simulink model "calibrate_imu_2_2"  (R2021b)
settings: Solver=VariableStepAuto  StartTime=0.0  StopTime=10.0  RelTol=1e-3
undefined symbols (not defined in the file or in its folder): X, Y, Z
libraries: nesl_utility x16, sm_lib x9, robotcorelib x1, aerolibnav x1
(part 2 of 2)

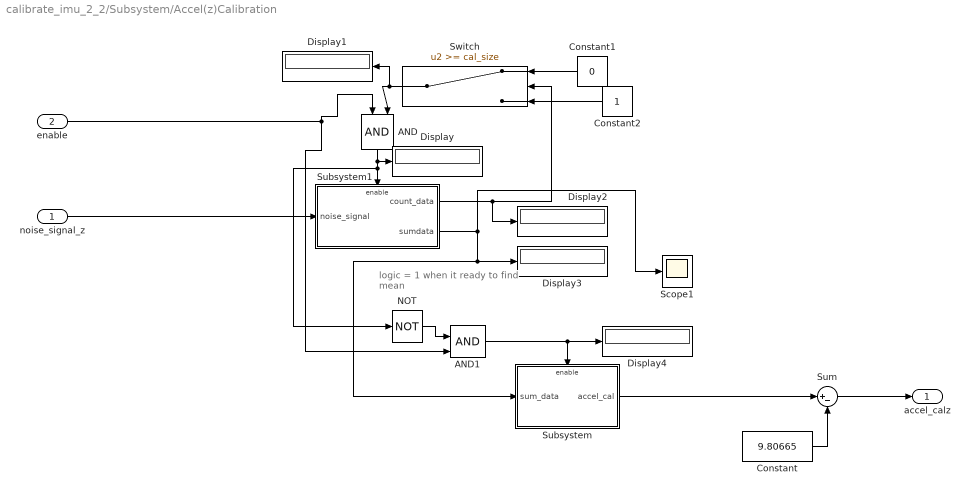
== system calibrate_imu_2_2/Subsystem/Accel(z)Calibration ==
  note: logic = 1 when it ready
      | to find mean
  noise_signal_z : Inport
  enable : Inport  Port=2
  AND : Logic  IconShape=distinctive  AllPortsSameDT=off  OutDataTypeStr=boolean
  AND1 : Logic  IconShape=distinctive  AllPortsSameDT=off  OutDataTypeStr=boolean
  Constant : Constant  Value=9.80665
  Constant1 : Constant  Value=0
  Constant2 : Constant
  Display{,1..4} (5 alike) : Display
  NOT : Logic  Operator=NOT  IconShape=distinctive  AllPortsSameDT=off  OutDataTypeStr=boolean
  Scope1 : Scope
  Subsystem : Subsystem
  Subsystem1 : Subsystem
  Sum : Sum  Inputs=|+-
  Switch : Switch  Threshold=cal_size
  accel_calz : Outport
  wires:
  Subsystem1/2(sumdata) -> Display3/1, Subsystem/1(sum_data), Scope1/1
  enable/1 -> AND/1, AND1/2
  Constant1/1 -> Switch/1
  Constant2/1 -> Switch/3
  Switch/1 -> Display1/1, AND/2
  AND/1 -> NOT/1, Subsystem1/Enable, Display/1
  NOT/1 -> AND1/1
  AND1/1 -> Subsystem/Enable, Display4/1
  Subsystem1/1(count_data) -> Switch/2, Display2/1
  noise_signal_z/1 -> Subsystem1/1(noise_signal)
  Sum/1 -> accel_calz/1
  Subsystem/1(accel_cal) -> Sum/1
  Constant/1 -> Sum/2

== system calibrate_imu_2_2/Gyro_Calibration/Gyro(x)Calibration/mean ==
  sum_data : Inport
  Enable : EnablePort
  Constant4 : Constant  Value=1000
  Divide : Product  Inputs=*/
  gyro_cal : Outport
  wires:
  Divide/1 -> gyro_cal/1  "gyro_cal"
  Constant4/1 -> Divide/2
  sum_data/1 -> Divide/1

== system calibrate_imu_2_2/Gyro_Calibration/Gyro(x)Calibration/sumdata ==
  noise_signal : Inport
  Enable : EnablePort
  Pulse Generator : DiscretePulseGenerator  PulseType=Time based  Period=sampleT  PulseWidth=5
  Subsystem : Subsystem
  count_data : Outport
  sumdata : Outport  Port=2
  wires:
  Pulse Generator/1 -> Subsystem/Trigger
  Subsystem/1(Out1) -> count_data/1
  Subsystem/2(Out2) -> sumdata/1
  noise_signal/1 -> Subsystem/1(noise signal)

== system calibrate_imu_2_2/Gyro_Calibration/Gyro(y)Calibration1/Subsystem ==
  sum_data : Inport
  Enable : EnablePort
  Constant4 : Constant  Value=1000
  Divide : Product  Inputs=*/
  gyro_cal : Outport
  wires:
  Divide/1 -> gyro_cal/1  "gyro_cal"
  Constant4/1 -> Divide/2
  sum_data/1 -> Divide/1

== system calibrate_imu_2_2/Gyro_Calibration/Gyro(y)Calibration1/Subsystem1 ==
  noise_signal : Inport
  Enable : EnablePort
  Pulse Generator : DiscretePulseGenerator  PulseType=Time based  Period=sampleT  PulseWidth=5
  Subsystem : Subsystem
  count_data : Outport
  sumdata : Outport  Port=2
  wires:
  Pulse Generator/1 -> Subsystem/Trigger
  Subsystem/1(Out1) -> count_data/1
  Subsystem/2(Out2) -> sumdata/1
  noise_signal/1 -> Subsystem/1(noise signal)

== system calibrate_imu_2_2/Gyro_Calibration/Gyro(z)Calibration2/Subsystem ==
  sum_data : Inport
  Enable : EnablePort
  Constant4 : Constant  Value=1000
  Divide : Product  Inputs=*/
  gyro_cal : Outport
  wires:
  Divide/1 -> gyro_cal/1  "gyro_cal"
  Constant4/1 -> Divide/2
  sum_data/1 -> Divide/1

== system calibrate_imu_2_2/Gyro_Calibration/Gyro(z)Calibration2/Subsystem1 ==
  noise_signal : Inport
  Enable : EnablePort
  Pulse Generator : DiscretePulseGenerator  PulseType=Time based  Period=sampleT  PulseWidth=5
  Subsystem : Subsystem
  count_data : Outport
  sumdata : Outport  Port=2
  wires:
  Pulse Generator/1 -> Subsystem/Trigger
  Subsystem/1(Out1) -> count_data/1
  Subsystem/2(Out2) -> sumdata/1
  noise_signal/1 -> Subsystem/1(noise signal)

== system calibrate_imu_2_2/Subsystem/Accel(x)Calibration/Subsystem ==
  sum_data : Inport
  Enable : EnablePort
  Constant4 : Constant  Value=1000
  Divide : Product  Inputs=*/
  accel_cal : Outport
  wires:
  Divide/1 -> accel_cal/1  "gyro_cal"
  Constant4/1 -> Divide/2
  sum_data/1 -> Divide/1

== system calibrate_imu_2_2/Subsystem/Accel(x)Calibration/Subsystem1 ==
  noise_signal : Inport
  Enable : EnablePort
  Pulse Generator : DiscretePulseGenerator  PulseType=Time based  Period=sampleT  PulseWidth=5
  Subsystem : Subsystem
  count_data : Outport
  sumdata : Outport  Port=2
  wires:
  Pulse Generator/1 -> Subsystem/Trigger
  Subsystem/1(Out1) -> count_data/1
  Subsystem/2(Out2) -> sumdata/1
  noise_signal/1 -> Subsystem/1(noise signal)

== system calibrate_imu_2_2/Subsystem/Accel(y)Calibration/Subsystem ==
  sum_data : Inport
  Enable : EnablePort
  Constant4 : Constant  Value=1000
  Divide : Product  Inputs=*/
  accel_cal : Outport
  wires:
  Divide/1 -> accel_cal/1  "gyro_cal"
  Constant4/1 -> Divide/2
  sum_data/1 -> Divide/1

== system calibrate_imu_2_2/Subsystem/Accel(y)Calibration/Subsystem1 ==
  noise_signal : Inport
  Enable : EnablePort
  Pulse Generator : DiscretePulseGenerator  PulseType=Time based  Period=sampleT  PulseWidth=5
  Subsystem : Subsystem
  count_data : Outport
  sumdata : Outport  Port=2
  wires:
  Pulse Generator/1 -> Subsystem/Trigger
  Subsystem/1(Out1) -> count_data/1
  Subsystem/2(Out2) -> sumdata/1
  noise_signal/1 -> Subsystem/1(noise signal)

== system calibrate_imu_2_2/Subsystem/Accel(z)Calibration/Subsystem ==
  sum_data : Inport
  Enable : EnablePort
  Constant4 : Constant  Value=1000
  Divide : Product  Inputs=*/
  accel_cal : Outport
  wires:
  Divide/1 -> accel_cal/1  "gyro_cal"
  Constant4/1 -> Divide/2
  sum_data/1 -> Divide/1

== system calibrate_imu_2_2/Subsystem/Accel(z)Calibration/Subsystem1 ==
  noise_signal : Inport
  Enable : EnablePort
  Pulse Generator : DiscretePulseGenerator  PulseType=Time based  Period=sampleT  PulseWidth=5
  Subsystem : Subsystem
  count_data : Outport
  sumdata : Outport  Port=2
  wires:
  Pulse Generator/1 -> Subsystem/Trigger
  Subsystem/1(Out1) -> count_data/1
  Subsystem/2(Out2) -> sumdata/1
  noise_signal/1 -> Subsystem/1(noise signal)

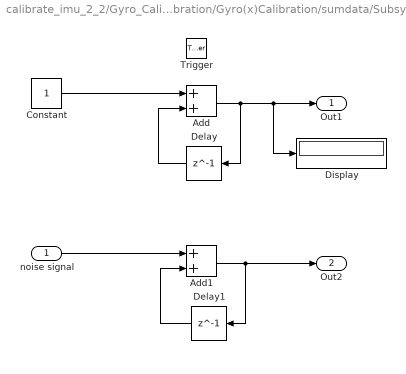
== system calibrate_imu_2_2/Gyro_Calibration/Gyro(x)Calibration/sumdata/Subsystem ==
  noise signal : Inport
  Trigger : TriggerPort  VariantControl=(inherit)  PortDimensions=1
  Add : Sum
  Add1 : Sum
  Constant : Constant
  Delay : Delay  DelayLength=1
  Delay1 : Delay  DelayLength=1
  Display : Display
  Out1 : Outport
  Out2 : Outport  Port=2
  wires:
  Add/1 -> Delay/1, Display/1, Out1/1
  Constant/1 -> Add/1
  Delay/1 -> Add/2
  Add1/1 -> Delay1/1, Out2/1
  Delay1/1 -> Add1/2
  noise signal/1 -> Add1/1

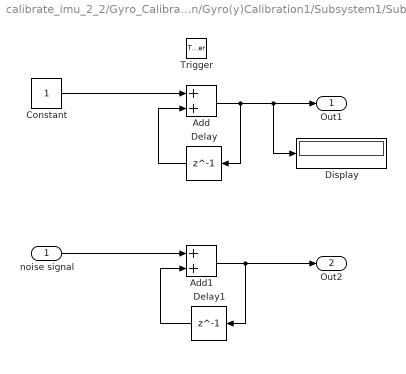
== system calibrate_imu_2_2/Gyro_Calibration/Gyro(y)Calibration1/Subsystem1/Subsystem ==
  noise signal : Inport
  Trigger : TriggerPort  VariantControl=(inherit)  PortDimensions=1
  Add : Sum
  Add1 : Sum
  Constant : Constant
  Delay : Delay  DelayLength=1
  Delay1 : Delay  DelayLength=1
  Display : Display
  Out1 : Outport
  Out2 : Outport  Port=2
  wires:
  Add/1 -> Delay/1, Display/1, Out1/1
  Constant/1 -> Add/1
  Delay/1 -> Add/2
  Add1/1 -> Delay1/1, Out2/1
  Delay1/1 -> Add1/2
  noise signal/1 -> Add1/1

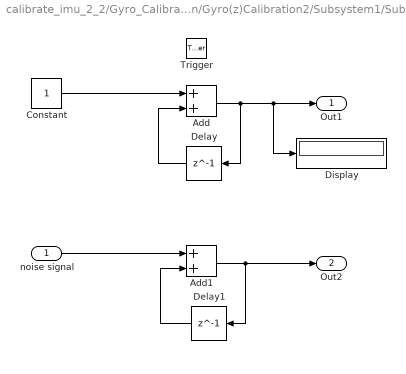
== system calibrate_imu_2_2/Gyro_Calibration/Gyro(z)Calibration2/Subsystem1/Subsystem ==
  noise signal : Inport
  Trigger : TriggerPort  VariantControl=(inherit)  PortDimensions=1
  Add : Sum
  Add1 : Sum
  Constant : Constant
  Delay : Delay  DelayLength=1
  Delay1 : Delay  DelayLength=1
  Display : Display
  Out1 : Outport
  Out2 : Outport  Port=2
  wires:
  Add/1 -> Delay/1, Display/1, Out1/1
  Constant/1 -> Add/1
  Delay/1 -> Add/2
  Add1/1 -> Delay1/1, Out2/1
  Delay1/1 -> Add1/2
  noise signal/1 -> Add1/1

== system calibrate_imu_2_2/Subsystem/Accel(x)Calibration/Subsystem1/Subsystem ==
  noise signal : Inport
  Trigger : TriggerPort  VariantControl=(inherit)  PortDimensions=1
  Add : Sum
  Add1 : Sum
  Constant : Constant
  Delay : Delay  DelayLength=1
  Delay1 : Delay  DelayLength=1
  Display : Display
  Out1 : Outport
  Out2 : Outport  Port=2
  wires:
  Add/1 -> Delay/1, Display/1, Out1/1
  Constant/1 -> Add/1
  Delay/1 -> Add/2
  Add1/1 -> Delay1/1, Out2/1
  Delay1/1 -> Add1/2
  noise signal/1 -> Add1/1

== system calibrate_imu_2_2/Subsystem/Accel(y)Calibration/Subsystem1/Subsystem ==
  noise signal : Inport
  Trigger : TriggerPort  VariantControl=(inherit)  PortDimensions=1
  Add : Sum
  Add1 : Sum
  Constant : Constant
  Delay : Delay  DelayLength=1
  Delay1 : Delay  DelayLength=1
  Display : Display
  Out1 : Outport
  Out2 : Outport  Port=2
  wires:
  Add/1 -> Delay/1, Display/1, Out1/1
  Constant/1 -> Add/1
  Delay/1 -> Add/2
  Add1/1 -> Delay1/1, Out2/1
  Delay1/1 -> Add1/2
  noise signal/1 -> Add1/1

== system calibrate_imu_2_2/Subsystem/Accel(z)Calibration/Subsystem1/Subsystem ==
  noise signal : Inport
  Trigger : TriggerPort  VariantControl=(inherit)  PortDimensions=1
  Add : Sum
  Add1 : Sum
  Constant : Constant
  Delay : Delay  DelayLength=1
  Delay1 : Delay  DelayLength=1
  Display : Display
  Out1 : Outport
  Out2 : Outport  Port=2
  wires:
  Add/1 -> Delay/1, Display/1, Out1/1
  Constant/1 -> Add/1
  Delay/1 -> Add/2
  Add1/1 -> Delay1/1, Out2/1
  Delay1/1 -> Add1/2
  noise signal/1 -> Add1/1
